simulink model "aufgabe3_sim"  (R2016b)
settings: Solver=VariableStepAuto  StartTime=0.0  StopTime=14  RelTol=1e-3
values from neighbouring files (symbols this model uses):
  A = double([0, 1, -1; -3411/62, -54163/28520, 1/1240;      6822/325, 1/3250, 54117/74750 - (7*1130385^(1/2))/7475])    [aufgabe1.m]    (also in aufgabe2.m; aufgabe3.m; aufgabe4.m; aufgabe5.m)
  bu = double([0; 12500/713; 0])    [aufgabe1.m]    (also in aufgabe2.m; aufgabe3.m; aufgabe4.m; aufgabe5.m)
  ct = [0 0 1]    [aufgabe1.m]    (also in aufgabe2.m; aufgabe3.m; aufgabe4.m; aufgabe5.m)
  kI = ke(4)    [aufgabe3.m]    (also in aufgabe4.m = 0.0065; aufgabe5.m = 0.0065)
  kP = 1/(ct*inv(eye(3)-phi)*gamma)    [aufgabe3.m]    (also in aufgabe4.m = 0.1488; aufgabe5.m = 0.1488)
  kx = kP*ct+ke(1:3)    [aufgabe3.m]    (also in aufgabe4.m = [-0.6050   -0.7335    0.3827]; aufgabe5.m = [-0.6050   -0.7335    0.3827])
  Ta = 10e-03    (= 0.01)    [aufgabe1.m]    (also in aufgabe2.m; aufgabe3.m; aufgabe4.m; aufgabe5.m)
libraries: simulink x1
settings Model: Creator=M  LastModifiedBy=M

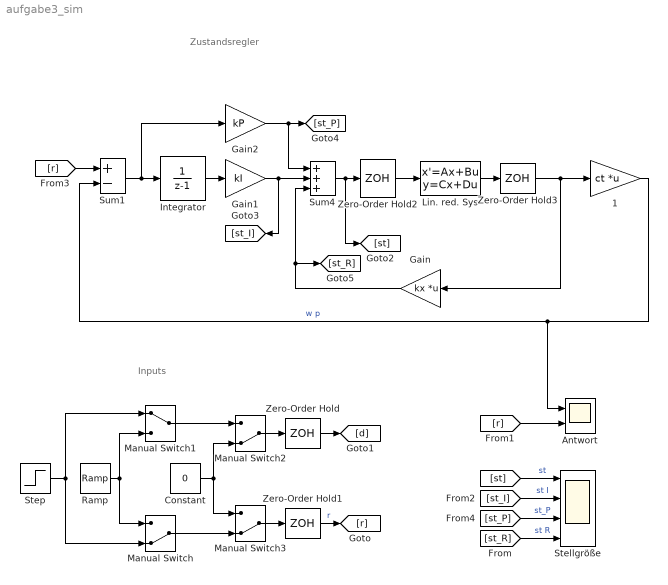
== system aufgabe3_sim ==
  note: Inputs
  note: Zustandsregler
  "   1" : Gain  Gain=ct  Multiplication=Matrix(K*u)
  Antwort : Scope  NumInputPorts=2
  Constant : Constant  Value=0
  Gain : Gain  Gain=kx  Multiplication=Matrix(K*u)  SampleTime=Ta
  Gain1 : Gain  Gain=kI
  Gain2 : Gain  Gain=kP
  Integrator : DiscreteTransferFcn  Denominator=[1 -1]  SampleTime=Ta
  Lin. red. Sys : StateSpace  A=A  B=bu  C=eye(3)  D=[0; 0 ; 0]  X0=[0,0,0]
  Manual Switch : ManualSwitch  CurrentSetting=0
  Manual Switch1 : ManualSwitch
  Manual Switch2 : ManualSwitch  CurrentSetting=0
  Manual Switch3 : ManualSwitch  CurrentSetting=0
  Ramp : simulink/Sources/Ramp  slope=1  start=1  X0=0
  Stellgröße : Scope  NumInputPorts=4
  Step : Step  SampleTime=0
  Sum1 : Sum  Inputs=+-
  Sum4 : Sum  Inputs=+++
  Zero-Order Hold : ZeroOrderHold  SampleTime=-1
  Zero-Order Hold1 : ZeroOrderHold  SampleTime=-1
  Zero-Order Hold2 : ZeroOrderHold  SampleTime=Ta
  Zero-Order Hold3 : ZeroOrderHold  SampleTime=Ta
  wires:
  Manual Switch1/1 -> Manual Switch2/1
  Constant/1 -> Manual Switch3/1, Manual Switch2/2
  Manual Switch2/1 -> Zero-Order Hold/1
  Manual Switch3/1 -> Zero-Order Hold1/1
  Manual Switch/1 -> Manual Switch3/2
  Ramp/1 -> Manual Switch/1, Manual Switch1/2
  Step/1 -> Manual Switch/2, Manual Switch1/1
  Zero-Order Hold1/1 -> [r]  "r"
  Zero-Order Hold/1 -> [d]
  Zero-Order Hold2/1 -> Lin. red. Sys/1
  Sum1/1 -> Gain2/1, Integrator/1
  Gain1/1 -> [st_I], Sum4/2
  Sum4/1 -> [st], Zero-Order Hold2/1
  Gain/1 -> [st_R], Sum4/3
  Lin. red. Sys/1 -> Zero-Order Hold3/1
  Zero-Order Hold3/1 -> Gain/1, "   1"/1
  [r] -> Antwort/2
  "   1"/1 -> Sum1/2, Antwort/1  "w p"
  Integrator/1 -> Gain1/1
  Gain2/1 -> [st_P], Sum4/1
  [r] -> Sum1/1
  [st] -> Stellgröße/1  "st"
  [st_I] -> Stellgröße/2  "st I"
  [st_P] -> Stellgröße/3  "st_P"
  [st_R] -> Stellgröße/4  "st R"
